simulink model "que_3"  (R2020b)
settings: Solver=VariableStepAuto  StartTime=0.0  StopTime=10.0  MaxStep=0.01  RelTol=1e-3
settings Model: Creator=Manasi  LastModifiedBy=Manasi

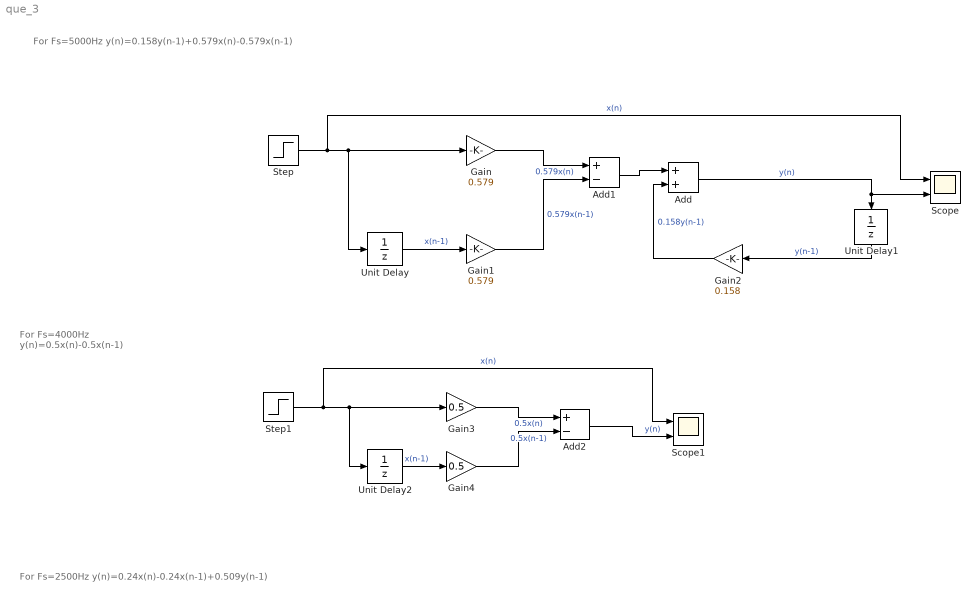
== system que_3 ==
  note: For Fs=5000Hz
      | y(n)=0.158y(n-1)+0.579x(n)-0.579x(n-1)
  note: For Fs=4000Hz
      | y(n)=0.5x(n)-0.5x(n-1)
  note: For Fs=2500Hz
      | y(n)=0.24x(n)-0.24x(n-1)+0.509y(n-1)
  Add : Sum
  Add1 : Sum  Inputs=+-
  Add2 : Sum  Inputs=+-
  Gain : Gain  Gain=0.579
  Gain1 : Gain  Gain=0.579
  Gain2 : Gain  Gain=0.158
  Gain3 : Gain  Gain=0.5
  Gain4 : Gain  Gain=0.5
  Scope : Scope  NumInputPorts=2
  Scope1 : Scope  NumInputPorts=2
  Step : Step  SampleTime=0
  Step1 : Step  SampleTime=0
  Unit Delay : UnitDelay  SampleTime=-1  HasFrameUpgradeWarning=on
  Unit Delay1 : UnitDelay  SampleTime=-1  HasFrameUpgradeWarning=on
  Unit Delay2 : UnitDelay  SampleTime=-1  HasFrameUpgradeWarning=on
  wires:
  Step/1 -> Scope/1, Unit Delay/1, Gain/1  "x(n)"
  Gain/1 -> Add1/1  "0.579x(n)"
  Unit Delay/1 -> Gain1/1  "x(n-1)"
  Gain1/1 -> Add1/2  "0.579x(n-1)"
  Add1/1 -> Add/1
  Add/1 -> Scope/2, Unit Delay1/1  "y(n)"
  Unit Delay1/1 -> Gain2/1  "y(n-1)"
  Gain2/1 -> Add/2  "0.158y(n-1)"
  Step1/1 -> Scope1/1, Unit Delay2/1, Gain3/1  "x(n)"
  Gain3/1 -> Add2/1  "0.5x(n)"
  Gain4/1 -> Add2/2  "0.5x(n-1)"
  Unit Delay2/1 -> Gain4/1  "x(n-1)"
  Add2/1 -> Scope1/2  "y(n)"
